simulink model "wtLinModelSimulink_LQI_2021a"  (R2021a)
settings: Solver=FixedStepAuto  StartTime=0.0  StopTime=1000  FixedStep=1/25  RelTol=1e-3
values from neighbouring files (symbols this model uses):
  Alqi = [Alqr		zeros(3,1) ... (first row only)    [wtLin_V164_8MW_V6_LQI.m]
  Alqr = sysNoFLC2.A    [wtLin_V164_8MW_V6_LQI.m]
  Bdlqi = [Bdlqr; 0]    [wtLin_V164_8MW_V6_LQI.m]
  Bdlqr = Blqr(:, distIndex)    [wtLin_V164_8MW_V6_LQI.m]
  Bulqi = [Bulqr; 0]    [wtLin_V164_8MW_V6_LQI.m]
  Bulqr = Blqr(:, distIndex+1:end)    [wtLin_V164_8MW_V6_LQI.m]
  Clqi = [Clqr	zeros(3,1)]    [wtLin_V164_8MW_V6_LQI.m]
  Clqr = sysNoFLC2.C    [wtLin_V164_8MW_V6_LQI.m]
  u_op = [simulationData(1,senIdx.Vhfree); simulationData(1,senIdx.pnt413); simulationData(1,senIdx.pfo017)]    [wtLin_V164_8MW_V6_LQI.m]
  x_bar_init = [py_init vy_init W_init]'    [wtLin_V164_8MW_V6_LQI.m]
  x_op_temp = [py_op vy_op W_op]'    [wtLin_V164_8MW_V6_LQI.m]
undefined symbols (not defined in the file or in its folder): Asys5, Bsys5, Csys5, Klqi, Klqr, x_bar_init_int, x_bar_init_sys5, x_op_temp_int, x_op_temp_sys5
settings Model: Creator=martin  LastModifiedBy=MROTR

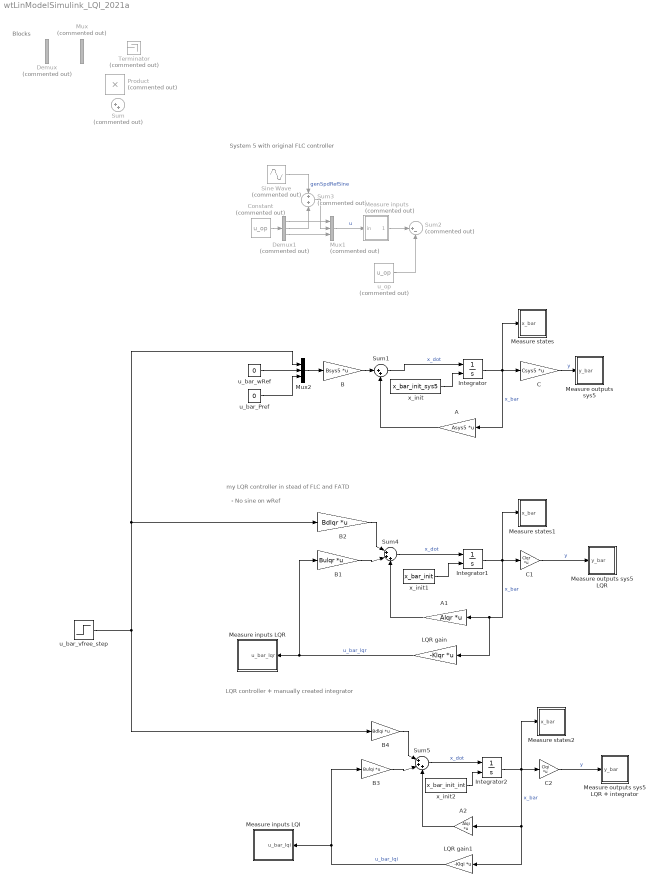
== system wtLinModelSimulink_LQI_2021a ==
  note: LQR controller + manually created integrator
  note: - No sine on wRef
  note: my LQR controller in stead of FLC and FATD
  note: System 5 with original FLC controller
  note: Blocks
  A : Gain  Gain=Asys5  Multiplication=Matrix(K*u)
  A1 : Gain  Gain=Alqr  Multiplication=Matrix(K*u)
  A2 : Gain  Gain=Alqi  Multiplication=Matrix(K*u)
  B : Gain  Gain=Bsys5  Multiplication=Matrix(K*u)
  B1 : Gain  Gain=Bulqr  Multiplication=Matrix(K*u)
  B2 : Gain  Gain=Bdlqr  Multiplication=Matrix(K*u)
  B3 : Gain  Gain=Bulqi  Multiplication=Matrix(K*u)
  B4 : Gain  Gain=Bdlqi  Multiplication=Matrix(K*u)
  C : Gain  Gain=Csys5  Multiplication=Matrix(K*u)
  C1 : Gain  Gain=Clqr  Multiplication=Matrix(K*u)
  C2 : Gain  Gain=Clqi  Multiplication=Matrix(K*u)
  Constant : Constant  Commented=on  Value=u_op
  Demux : Demux  Commented=on  Outputs=2
  Demux1 : Demux  Commented=on  Outputs=3
  Integrator : Integrator  InitialConditionSource=external
  Integrator1 : Integrator  InitialConditionSource=external
  Integrator2 : Integrator  InitialConditionSource=external
  LQR gain : Gain  Gain=-Klqr  Multiplication=Matrix(K*u)
  LQR gain1 : Gain  Gain=-Klqi  Multiplication=Matrix(K*u)
  Measure inputs : Subsystem  Commented=on
  Measure inputs LQI : Subsystem
  Measure inputs LQR : Subsystem
  Measure outputs sys5 : Subsystem
  Measure outputs sys5 LQR : Subsystem
  Measure outputs sys5 LQR + integrator : Subsystem
  Measure states : Subsystem
  Measure states1 : Subsystem
  Measure states2 : Subsystem
  Mux : Mux  Commented=on  Inputs=2
  Mux1 : Mux  Commented=on  Inputs=3
  Mux2 : Mux  Inputs=3
  Product : Product  Commented=on
  Sine Wave : Sin  Commented=on  Amplitude=20  Frequency=0.6302  SampleTime=0
  Sum : Sum  Commented=on  Inputs=|++
  Sum1 : Sum  Inputs=|++
  Sum2 : Sum  Commented=on  Inputs=|+-
  Sum3 : Sum  Commented=on  Inputs=+|+
  Sum4 : Sum  Inputs=|+++
  Sum5 : Sum  Inputs=|+++
  Terminator : Terminator  Commented=on
  u_bar_Pref : Constant  Value=0
  u_bar_vfree_step : Step  Time=300  SampleTime=0
  u_bar_wRef : Constant  Value=0
  u_op : Constant  Commented=on  Value=u_op
  x_init : Constant  Value=x_bar_init_sys5
  x_init1 : Constant  Value=x_bar_init
  x_init2 : Constant  Value=x_bar_init_int
  wires:
  A/1 -> Sum1/2
  Sum1/1 -> Integrator/1  "x_dot"
  B/1 -> Sum1/1
  Mux1/1 -> Measure inputs/1(in)  "u"
  x_init/1 -> Integrator/2
  Integrator/1 -> Measure states/1(x_bar), C/1, A/1  "x_bar"
  Measure inputs/1(out) -> Sum2/1
  C/1 -> Measure outputs sys5/1(y_bar)  "y"
  u_op/1 -> Sum2/2
  Constant/1 -> Demux1/1
  Demux1/2 -> Sum3/2
  Sine Wave/1 -> Sum3/1  "genSpdRefSine"
  Demux1/1 -> Mux1/1
  Demux1/3 -> Mux1/3
  Sum3/1 -> Mux1/2
  C1/1 -> Measure outputs sys5 LQR/1(y_bar)  "y"
  Integrator1/1 -> Measure states1/1(x_bar), C1/1, LQR gain/1, A1/1  "x_bar"
  A1/1 -> Sum4/3
  LQR gain/1 -> B1/1, Measure inputs LQR/1(u_bar_lqr)  "u_bar_lqr"
  x_init1/1 -> Integrator1/2
  Sum4/1 -> Integrator1/1  "x_dot"
  B1/1 -> Sum4/2
  B2/1 -> Sum4/1
  LQR gain1/1 -> Measure inputs LQI/1(u_bar_lqi), B3/1  "u_bar_lqi"
  Integrator2/1 -> Measure states2/1(x_bar), C2/1, LQR gain1/1, A2/1  "x_bar"
  x_init2/1 -> Integrator2/2
  Sum5/1 -> Integrator2/1  "x_dot"
  B4/1 -> Sum5/1
  B3/1 -> Sum5/2
  A2/1 -> Sum5/3
  C2/1 -> Measure outputs sys5 LQR + integrator/1(y_bar)  "y"
  u_bar_wRef/1 -> Mux2/2
  u_bar_vfree_step/1 -> B4/1, B2/1, Mux2/1
  u_bar_Pref/1 -> Mux2/3
  Mux2/1 -> B/1

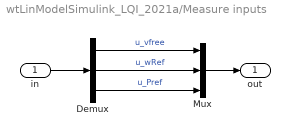
== system wtLinModelSimulink_LQI_2021a/Measure inputs ==
  in : Inport
  Demux : Demux  Outputs=3
  Mux : Mux  Inputs=3
  out : Outport
  wires:
  Demux/1 -> Mux/1  "u_vfree"
  Demux/2 -> Mux/2  "u_wRef"
  Demux/3 -> Mux/3  "u_Pref"
  Mux/1 -> out/1
  in/1 -> Demux/1

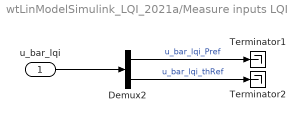
== system wtLinModelSimulink_LQI_2021a/Measure inputs LQI ==
  u_bar_lqi : Inport
  Demux2 : Demux  Outputs=2
  Terminator1 : Terminator
  Terminator2 : Terminator
  wires:
  Demux2/1 -> Terminator1/1  "u_bar_lqi_Pref"
  Demux2/2 -> Terminator2/1  "u_bar_lqi_thRef"
  u_bar_lqi/1 -> Demux2/1

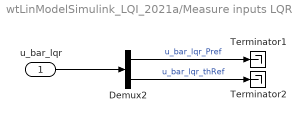
== system wtLinModelSimulink_LQI_2021a/Measure inputs LQR ==
  u_bar_lqr : Inport
  Demux2 : Demux  Outputs=2
  Terminator1 : Terminator
  Terminator2 : Terminator
  wires:
  Demux2/1 -> Terminator1/1  "u_bar_lqr_Pref"
  Demux2/2 -> Terminator2/1  "u_bar_lqr_thRef"
  u_bar_lqr/1 -> Demux2/1

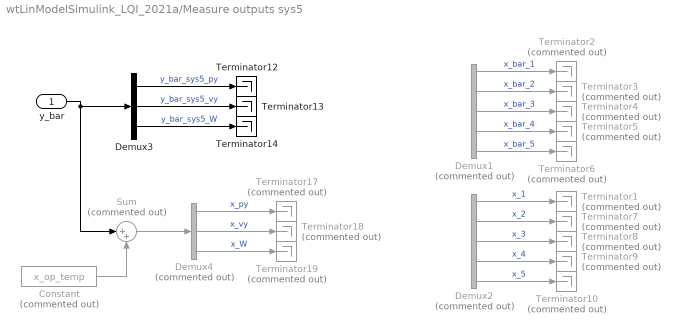
== system wtLinModelSimulink_LQI_2021a/Measure outputs sys5 ==
  y_bar : Inport
  Constant : Constant  Commented=on  Value=x_op_temp
  Demux1 : Demux  Commented=on  Outputs=5
  Demux2 : Demux  Commented=on  Outputs=5
  Demux3 : Demux  Outputs=3
  Demux4 : Demux  Commented=on  Outputs=3
  Sum : Sum  Commented=on  Inputs=|++
  Terminator{1..10,17..19} (13 alike) : Terminator  Commented=on
  Terminator12 : Terminator
  Terminator13 : Terminator
  Terminator14 : Terminator
  wires:
  y_bar/1 -> Sum/1, Demux3/1
  Constant/1 -> Sum/2
  Demux3/3 -> Terminator14/1  "y_bar_sys5_W"
  Demux3/1 -> Terminator12/1  "y_bar_sys5_py"
  Demux3/2 -> Terminator13/1  "y_bar_sys5_vy"
  Demux4/2 -> Terminator18/1  "x_vy"
  Demux4/3 -> Terminator19/1  "x_W"
  Demux4/1 -> Terminator17/1  "x_py"
  Demux1/4 -> Terminator5/1  "x_bar_4"
  Demux1/2 -> Terminator3/1  "x_bar_2"
  ? -> Demux1/1
  Demux1/3 -> Terminator4/1  "x_bar_3"
  Demux1/5 -> Terminator6/1  "x_bar_5"
  Demux1/1 -> Terminator2/1  "x_bar_1"
  Demux2/3 -> Terminator8/1  "x_3"
  Demux2/5 -> Terminator10/1  "x_5"
  Demux2/4 -> Terminator9/1  "x_4"
  ? -> Demux2/1
  Demux2/1 -> Terminator1/1  "x_1"
  Demux2/2 -> Terminator7/1  "x_2"
  Sum/1 -> Demux4/1

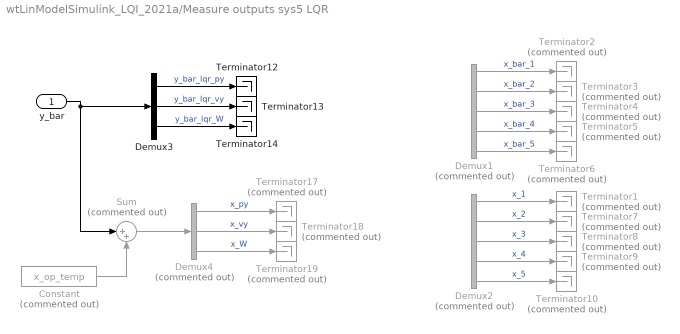
== system wtLinModelSimulink_LQI_2021a/Measure outputs sys5 LQR ==
  y_bar : Inport
  Constant : Constant  Commented=on  Value=x_op_temp
  Demux1 : Demux  Commented=on  Outputs=5
  Demux2 : Demux  Commented=on  Outputs=5
  Demux3 : Demux  Outputs=3
  Demux4 : Demux  Commented=on  Outputs=3
  Sum : Sum  Commented=on  Inputs=|++
  Terminator{1..10,17..19} (13 alike) : Terminator  Commented=on
  Terminator12 : Terminator
  Terminator13 : Terminator
  Terminator14 : Terminator
  wires:
  y_bar/1 -> Sum/1, Demux3/1
  Constant/1 -> Sum/2
  Demux3/3 -> Terminator14/1  "y_bar_lqr_W"
  Demux3/1 -> Terminator12/1  "y_bar_lqr_py"
  Demux3/2 -> Terminator13/1  "y_bar_lqr_vy"
  Demux4/2 -> Terminator18/1  "x_vy"
  Demux4/3 -> Terminator19/1  "x_W"
  Demux4/1 -> Terminator17/1  "x_py"
  Demux1/4 -> Terminator5/1  "x_bar_4"
  Demux1/2 -> Terminator3/1  "x_bar_2"
  ? -> Demux1/1
  Demux1/3 -> Terminator4/1  "x_bar_3"
  Demux1/5 -> Terminator6/1  "x_bar_5"
  Demux1/1 -> Terminator2/1  "x_bar_1"
  Demux2/3 -> Terminator8/1  "x_3"
  Demux2/5 -> Terminator10/1  "x_5"
  Demux2/4 -> Terminator9/1  "x_4"
  ? -> Demux2/1
  Demux2/1 -> Terminator1/1  "x_1"
  Demux2/2 -> Terminator7/1  "x_2"
  Sum/1 -> Demux4/1

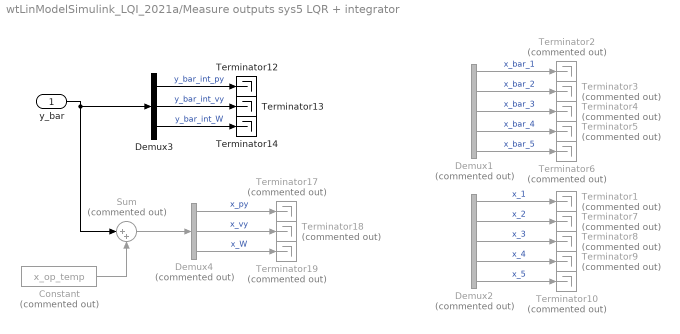
== system wtLinModelSimulink_LQI_2021a/Measure outputs sys5 LQR + integrator ==
  y_bar : Inport
  Constant : Constant  Commented=on  Value=x_op_temp
  Demux1 : Demux  Commented=on  Outputs=5
  Demux2 : Demux  Commented=on  Outputs=5
  Demux3 : Demux  Outputs=3
  Demux4 : Demux  Commented=on  Outputs=3
  Sum : Sum  Commented=on  Inputs=|++
  Terminator{1..10,17..19} (13 alike) : Terminator  Commented=on
  Terminator12 : Terminator
  Terminator13 : Terminator
  Terminator14 : Terminator
  wires:
  y_bar/1 -> Sum/1, Demux3/1
  Constant/1 -> Sum/2
  Demux3/3 -> Terminator14/1  "y_bar_int_W"
  Demux3/1 -> Terminator12/1  "y_bar_int_py"
  Demux3/2 -> Terminator13/1  "y_bar_int_vy"
  Demux4/2 -> Terminator18/1  "x_vy"
  Demux4/3 -> Terminator19/1  "x_W"
  Demux4/1 -> Terminator17/1  "x_py"
  Demux1/4 -> Terminator5/1  "x_bar_4"
  Demux1/2 -> Terminator3/1  "x_bar_2"
  ? -> Demux1/1
  Demux1/3 -> Terminator4/1  "x_bar_3"
  Demux1/5 -> Terminator6/1  "x_bar_5"
  Demux1/1 -> Terminator2/1  "x_bar_1"
  Demux2/3 -> Terminator8/1  "x_3"
  Demux2/5 -> Terminator10/1  "x_5"
  Demux2/4 -> Terminator9/1  "x_4"
  ? -> Demux2/1
  Demux2/1 -> Terminator1/1  "x_1"
  Demux2/2 -> Terminator7/1  "x_2"
  Sum/1 -> Demux4/1

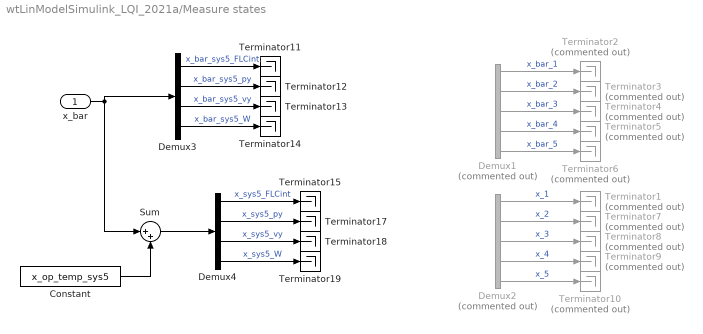
== system wtLinModelSimulink_LQI_2021a/Measure states ==
  x_bar : Inport
  Constant : Constant  Value=x_op_temp_sys5
  Demux1 : Demux  Commented=on  Outputs=5
  Demux2 : Demux  Commented=on  Outputs=5
  Demux3 : Demux
  Demux4 : Demux
  Sum : Sum  Inputs=|++
  Terminator{1..10} (10 alike) : Terminator  Commented=on
  Terminator{11..15,17..19} (8 alike) : Terminator
  wires:
  x_bar/1 -> Sum/1, Demux3/1
  Constant/1 -> Sum/2
  Demux3/4 -> Terminator14/1  "x_bar_sys5_W"
  Demux3/2 -> Terminator12/1  "x_bar_sys5_py"
  Demux3/3 -> Terminator13/1  "x_bar_sys5_vy"
  Demux3/1 -> Terminator11/1  "x_bar_sys5_FLCint"
  Demux4/3 -> Terminator18/1  "x_sys5_vy"
  Demux4/4 -> Terminator19/1  "x_sys5_W"
  Demux4/1 -> Terminator15/1  "x_sys5_FLCint"
  Demux4/2 -> Terminator17/1  "x_sys5_py"
  Demux1/4 -> Terminator5/1  "x_bar_4"
  Demux1/2 -> Terminator3/1  "x_bar_2"
  ? -> Demux1/1
  Demux1/3 -> Terminator4/1  "x_bar_3"
  Demux1/5 -> Terminator6/1  "x_bar_5"
  Demux1/1 -> Terminator2/1  "x_bar_1"
  Demux2/3 -> Terminator8/1  "x_3"
  Demux2/5 -> Terminator10/1  "x_5"
  Demux2/4 -> Terminator9/1  "x_4"
  ? -> Demux2/1
  Demux2/1 -> Terminator1/1  "x_1"
  Demux2/2 -> Terminator7/1  "x_2"
  Sum/1 -> Demux4/1

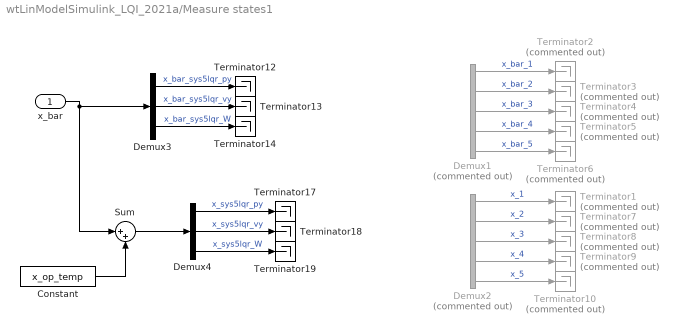
== system wtLinModelSimulink_LQI_2021a/Measure states1 ==
  x_bar : Inport
  Constant : Constant  Value=x_op_temp
  Demux1 : Demux  Commented=on  Outputs=5
  Demux2 : Demux  Commented=on  Outputs=5
  Demux3 : Demux  Outputs=3
  Demux4 : Demux  Outputs=3
  Sum : Sum  Inputs=|++
  Terminator{1..10} (10 alike) : Terminator  Commented=on
  Terminator{12..14,17..19} (6 alike) : Terminator
  wires:
  x_bar/1 -> Sum/1, Demux3/1
  Constant/1 -> Sum/2
  Demux3/3 -> Terminator14/1  "x_bar_sys5lqr_W"
  Demux3/1 -> Terminator12/1  "x_bar_sys5lqr_py"
  Demux3/2 -> Terminator13/1  "x_bar_sys5lqr_vy"
  Demux4/2 -> Terminator18/1  "x_sys5lqr_vy"
  Demux4/3 -> Terminator19/1  "x_sys5lqr_W"
  Demux4/1 -> Terminator17/1  "x_sys5lqr_py"
  Demux1/4 -> Terminator5/1  "x_bar_4"
  Demux1/2 -> Terminator3/1  "x_bar_2"
  ? -> Demux1/1
  Demux1/3 -> Terminator4/1  "x_bar_3"
  Demux1/5 -> Terminator6/1  "x_bar_5"
  Demux1/1 -> Terminator2/1  "x_bar_1"
  Demux2/3 -> Terminator8/1  "x_3"
  Demux2/5 -> Terminator10/1  "x_5"
  Demux2/4 -> Terminator9/1  "x_4"
  ? -> Demux2/1
  Demux2/1 -> Terminator1/1  "x_1"
  Demux2/2 -> Terminator7/1  "x_2"
  Sum/1 -> Demux4/1

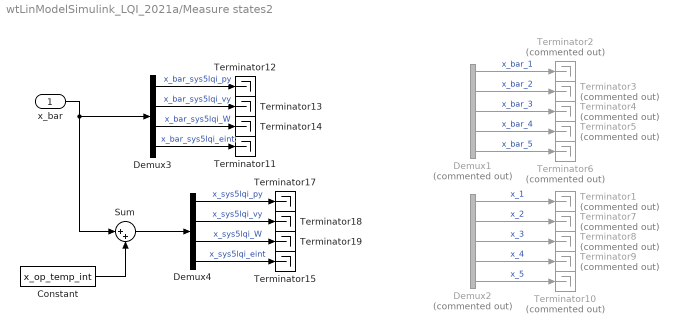
== system wtLinModelSimulink_LQI_2021a/Measure states2 ==
  x_bar : Inport
  Constant : Constant  Value=x_op_temp_int
  Demux1 : Demux  Commented=on  Outputs=5
  Demux2 : Demux  Commented=on  Outputs=5
  Demux3 : Demux
  Demux4 : Demux
  Sum : Sum  Inputs=|++
  Terminator{1..10} (10 alike) : Terminator  Commented=on
  Terminator{11..15,17..19} (8 alike) : Terminator
  wires:
  x_bar/1 -> Sum/1, Demux3/1
  Constant/1 -> Sum/2
  Demux3/3 -> Terminator14/1  "x_bar_sys5lqi_W"
  Demux3/1 -> Terminator12/1  "x_bar_sys5lqi_py"
  Demux3/2 -> Terminator13/1  "x_bar_sys5lqi_vy"
  Demux4/2 -> Terminator18/1  "x_sys5lqi_vy"
  Demux4/3 -> Terminator19/1  "x_sys5lqi_W"
  Demux4/1 -> Terminator17/1  "x_sys5lqi_py"
  Demux1/4 -> Terminator5/1  "x_bar_4"
  Demux1/2 -> Terminator3/1  "x_bar_2"
  ? -> Demux1/1
  Demux1/3 -> Terminator4/1  "x_bar_3"
  Demux1/5 -> Terminator6/1  "x_bar_5"
  Demux1/1 -> Terminator2/1  "x_bar_1"
  Demux2/3 -> Terminator8/1  "x_3"
  Demux2/5 -> Terminator10/1  "x_5"
  Demux2/4 -> Terminator9/1  "x_4"
  ? -> Demux2/1
  Demux2/1 -> Terminator1/1  "x_1"
  Demux2/2 -> Terminator7/1  "x_2"
  Sum/1 -> Demux4/1
  Demux4/4 -> Terminator15/1  "x_sys5lqi_eint"
  Demux3/4 -> Terminator11/1  "x_bar_sys5lqi_eint"
